simulink model "Kinematic_sim"  (R2022b)
settings: Solver=VariableStepAuto  StartTime=0.0  StopTime=10.0  RelTol=1e-3
values from neighbouring files (symbols this model uses):
  d1 = 150    [Kinematic.m]
  d2 = 40    [Kinematic.m]
  l1 = 544    [Kinematic.m]
  l2 = 575    [Kinematic.m]
  l3 = 675    [Kinematic.m]
  l4 = 90    [Kinematic.m]
settings Model: Creator=nhan  LastModifiedBy=nhan

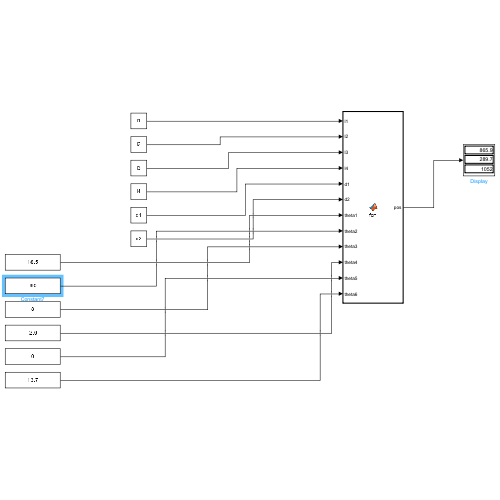
[thumbnail: Simulink's stored preview of the top-level diagram]
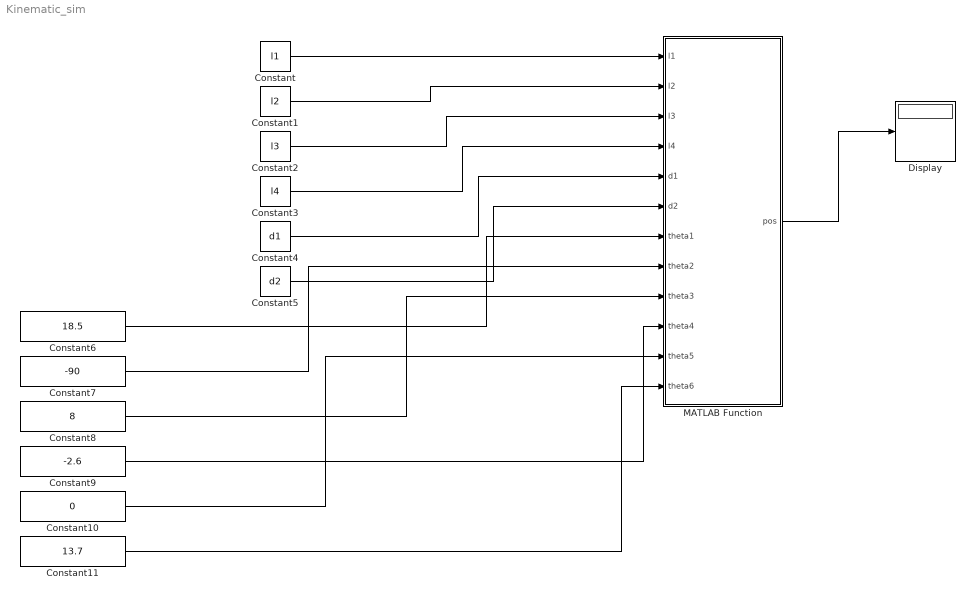
== system Kinematic_sim ==
  Constant : Constant  Value=l1
  Constant1 : Constant  Value=l2
  Constant10 : Constant  Value=0
  Constant11 : Constant  Value=13.7
  Constant2 : Constant  Value=l3
  Constant3 : Constant  Value=l4
  Constant4 : Constant  Value=d1
  Constant5 : Constant  Value=d2
  Constant6 : Constant  Value=18.5
  Constant7 : Constant  Value=-90
  Constant8 : Constant  Value=8
  Constant9 : Constant  Value=-2.6
  Display : Display
  MATLAB Function : MATLAB Function  TreatAsAtomicUnit=on
  wires:
  Constant/1 -> MATLAB Function/1(l1)
  Constant1/1 -> MATLAB Function/2(l2)
  Constant2/1 -> MATLAB Function/3(l3)
  Constant3/1 -> MATLAB Function/4(l4)
  Constant4/1 -> MATLAB Function/5(d1)
  Constant5/1 -> MATLAB Function/6(d2)
  Constant6/1 -> MATLAB Function/7(theta1)
  Constant7/1 -> MATLAB Function/8(theta2)
  Constant8/1 -> MATLAB Function/9(theta3)
  Constant9/1 -> MATLAB Function/10(theta4)
  Constant10/1 -> MATLAB Function/11(theta5)
  Constant11/1 -> MATLAB Function/12(theta6)
  MATLAB Function/1(pos) -> Display/1

== matlab function Kinematic_sim/MATLAB Function ==
  data: l1 input; pos output; l2 input; l3 input; l4 input; d1 input; d2 input; theta1 input; theta2 input; theta3 input; theta4 input; theta5 input; theta6 input
function pos = fcn(l1, l2, l3, l4, d1, d2, theta1, theta2, theta3, theta4, theta5, theta6)

c1 = cosd(theta1); s1 = sind(theta1);
c2 = cosd(theta2); s2=sind(theta2);
c4 = cosd(theta4); s4 = sind(theta4);
c5 = cosd(theta5); s5 = sind(theta5);
s2_3 = sind(theta2 + theta3);
c2_3 = cosd(theta2 + theta3);

% Công thức tính Px, Py, Pz
Px = -l4 * s5 * (c1 * c4 * c2_3 + s1 * s4) - l4 * c5 * c1 * s2_3 + d2 * c1 * c2_3 - l3 * c1 * s2_3 + c1 * (l2 * c2 + d1);
Py = -l4 * s5 * (s1 * c4 * c2_3 - c1 * s4) - l4 * c5 * s1 * s2_3 + d2 * s1 * c2_3 - l3 * s1 * s2_3 + s1 * (l2 * c2 + d1);
Pz = l4 * s5 * c4 * s2_3 - l4 * c5 * c2_3 - d2 * s2_3 - l3 * c2_3 + l1 - l2 * s2;
pos=[Px;Py;Pz];
